simulink model "springMassDamperSystem"  (R2024a)
settings: Solver=ode45  StartTime=0.0  StopTime=20  MaxStep=0.01  RelTol=1e-3
values from neighbouring files (symbols this model uses):
  c = 2000    [systemParameters1.m]
  k = 10000    [systemParameters1.m]
  m = 100    [systemParameters1.m]
settings Model: Creator=Sarthak Sahoo  LastModifiedBy=Sarthak Sahoo
settings SolverCC: ZeroCrossAlgorithm=Adaptive
settings RTWCC: GPUComputeCapability=3.5

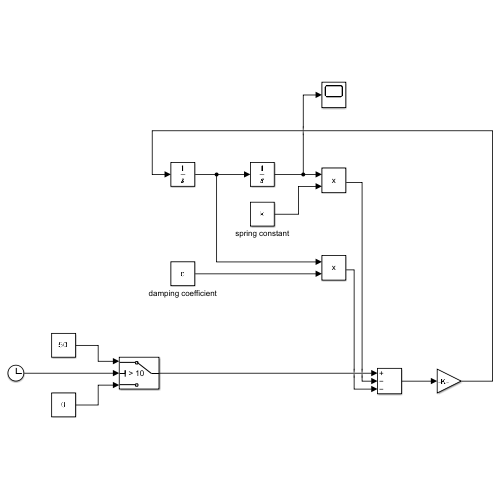
[thumbnail: Simulink's stored preview of the top-level diagram]
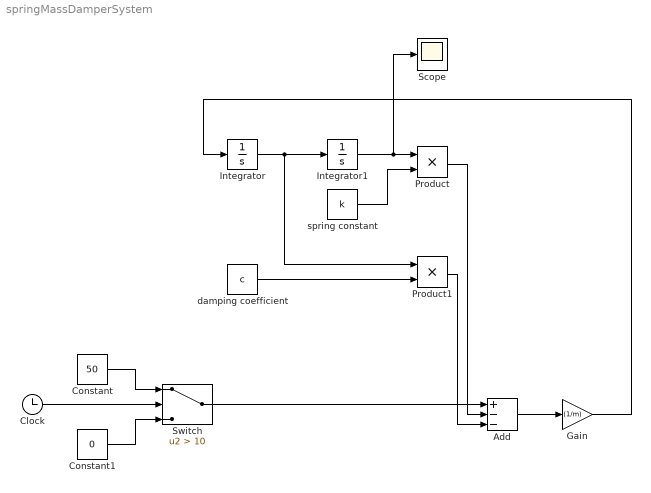
== system springMassDamperSystem ==
  Add : Sum  Inputs=+--
  Clock : Clock
  Constant : Constant  Value=50
  Constant1 : Constant  Value=0
  Gain : Gain  Gain=(1/m)
  Integrator : Integrator
  Integrator1 : Integrator
  Product : Product
  Product1 : Product
  Scope : Scope
  Switch : Switch  Criteria=u2 > Threshold  Threshold=10  SaturateOnIntegerOverflow=off  InputSameDT=off
  damping coefficient : Constant  Value=c
  spring constant : Constant  Value=k
  wires:
  Integrator/1 -> Product1/1, Integrator1/1
  Integrator1/1 -> Scope/1, Product/1
  spring constant/1 -> Product/2
  damping coefficient/1 -> Product1/2
  Constant/1 -> Switch/1
  Constant1/1 -> Switch/3
  Clock/1 -> Switch/2
  Switch/1 -> Add/1
  Product/1 -> Add/2
  Product1/1 -> Add/3
  Add/1 -> Gain/1
  Gain/1 -> Integrator/1
